simulink model "ws2opc_m"  (Simulink 8.5)
settings: Solver=ode45  SolverMode=SingleTasking  StartTime=0.0  StopTime=999999  MaxStep=10  RelTol=1e-3  AbsTol=1e-3
values from neighbouring files (symbols this model uses):
  U = st_Varia('LongNames')    [ws2opc_i.m]
  x0 = zeros(length(P.WSInputNames)+1,1)    [opc2ws_s.m]    (also in ws2opc_i.m = []; ws2opc_s.m = [])
undefined symbols (not defined in the file or in its folder): B
settings Model: Creator=M.Sparnaaij  LastModifiedBy=Martijn
settings DataIOCC: LimitDataPoints=off  SaveOutput=off  SaveTime=off  SignalLoggingName=sigsOut
settings OptimizationCC: BooleanDataType=off
settings DebuggingCC: SaveWithParameterizedLinksMsg=none  SignalResolutionControl=TryResolveAllWithWarning  MultiTaskDSMMsg=warning  MultiTaskCondExecSysMsg=none  FcnCallInpInsideContextMsg=EnableAllAsWarning  StrictBusMsg=None
settings HardwareCC: TargetUnknown=on

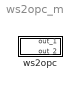
== system ws2opc_m ==
  ws2opc : Subsystem  Description=ws2opc
      mask init:
      | filenaam='./StimelaData/WSInterface.mat';
      | 
      | [Pn,Fn,Fext]=Fileprop(filenaam);
      | 
      | errstr = st_UniqName(filenaam,'filenaam=''','SubSystem','OpenFcn');
      | if errstr, error([errstr 'The filename "' filenaam '" is already in use. Choose a different filename.']), end
      | 
      | [B,x0,U]=ws2opc_i(filenaam);
      | P = ws2opc_p(filenaam);
      settings: OpenFcn=|
      | filenaam='./StimelaData/WSInterface.mat';
      | st_ParameterInput('init',gcb,filenaam,'ws2opc');
      mask Display:
      | plot(0,0,100,100,[80 100],[ 80 80],[80 100],[ 20 20])
      | patch([20 80 80 20 20],[10 10 90  90 10],[1 0 0])
      | text(50,50,'ws', 'horizontalAlignment', 'center', 'verticalAlignment', 'middle');
      | disp('')

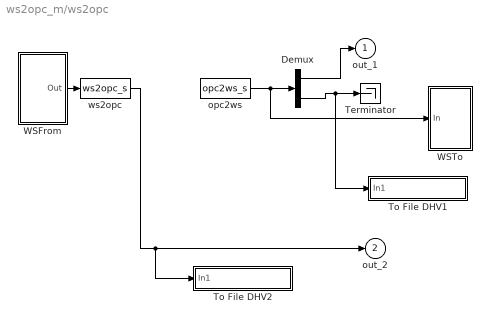
== system ws2opc_m/ws2opc ==
  Demux : Demux  Outputs=[1 -1]
  Terminator : Terminator
  To File DHV1 : Subsystem  mask(To File DHV){naam=[filenaam(1:length(filenaam)-4) '_ES.sti']}
      mask prompts: naam "Naam van bestand"
      mask init:
      | set_param([gcb '/To File'],'Filename',naam);
      mask Display: disp(naam)
  To File DHV2 : Subsystem  mask(To File DHV){naam=[filenaam(1:length(filenaam)-4) '_EM.sti']}
      mask prompts: naam "Naam van bestand"
      mask init:
      | set_param([gcb '/To File'],'Filename',naam);
      mask Display: disp(naam)
  WSFrom : Subsystem
  WSTo : Subsystem
  opc2ws : S-Function  FunctionName=opc2ws_s  Parameters=B,x0,U,P
  ws2opc : S-Function  FunctionName=ws2opc_s  Parameters=B,x0,U,P
  out_1 : Outport  InitialOutput=0
  out_2 : Outport  Port=2  InitialOutput=0
  wires:
  Demux/1 -> out_1/1
  opc2ws/1 -> Demux/1, WSTo/1(In)
  Demux/2 -> Terminator/1, To File DHV1/1(In1)
  WSFrom/1(Out) -> ws2opc/1
  ws2opc/1 -> out_2/1, To File DHV2/1(In1)

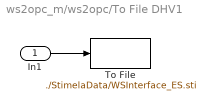
== system ws2opc_m/ws2opc/To File DHV1 ==
  In1 : Inport
  To File : ToFile  Filename=./StimelaData/WSInterface_ES.sti  MatrixName=ws2opcES
  wires:
  In1/1 -> To File/1

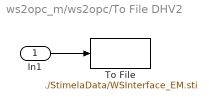
== system ws2opc_m/ws2opc/To File DHV2 ==
  In1 : Inport
  To File : ToFile  Filename=./StimelaData/WSInterface_EM.sti  MatrixName=ws2opcEM
  wires:
  In1/1 -> To File/1

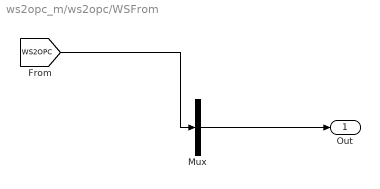
== system ws2opc_m/ws2opc/WSFrom ==
  Mux : Mux  Inputs=1
  Out : Outport
  wires:
  Mux/1 -> Out/1
  [WS2OPC] -> Mux/1

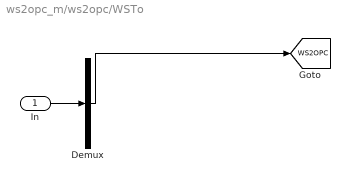
== system ws2opc_m/ws2opc/WSTo ==
  In : Inport
  Demux : Demux  Outputs=1
  tag scope: WS2OPC=global
  wires:
  In/1 -> Demux/1
  Demux/1 -> [WS2OPC]
